simulink model "untitled_org"  (Simulink 10.0)
settings: Solver=ode45  StartTime=0.0  StopTime=10.0  RelTol=1e-3  EnableMultiTasking=on
undefined symbols (not defined in the file): water_level
libraries: nesl_utility x8, sm_lib x3
settings Model: Creator=Metti  LastModifiedBy=bhisma
settings DataIOCC: LimitDataPoints=on
settings OptimizationCC: ExpressionDepthLimit=2147483647
settings DebuggingCC: SolverPrmCheckMsg=warning  StateNameClashWarn=warning
settings GRTTargetCC: GeneratePreprocessorConditionals=Disable all  CombineOutputUpdateFcns=on  GRTInterface=off
settings ConfigComp: CovExternalEMLEnable=off
settings SimscapeCC: SimscapeNormalizeSystem=off
settings ConfigurationSet: Description=SimMechanics 2G

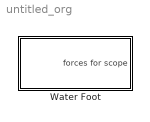
== system untitled_org ==
  Water Foot : Subsystem  AncestorBlock=WaterRunner_lib/Water Foot

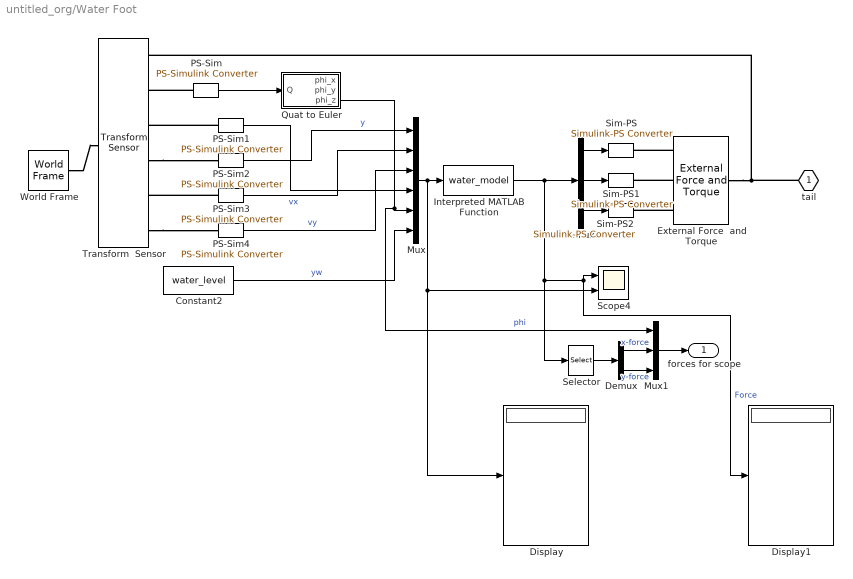
== system untitled_org/Water Foot ==
  Constant2 : Constant  Value=water_level
  Demux : Demux  Outputs=2
  Demux1 : Demux  Outputs=3
  Display : Display
  Display1 : Display
  External Force  and Torque : sm_lib/Forces and Torques/External Force and Torque  ForceResolutionFrame=World  EnableForceX=off  EnableForceY=on  EnableForceZ=on  EnableForce=off  TorqueResolutionFrame=World  EnableTorqueX=on  EnableTorqueY=off  EnableTorqueZ=off  EnableTorque=off
  Interpreted MATLAB Function : MATLABFcn  MATLABFcn=water_model
  Mux : Mux  Inputs=6
  Mux1 : Mux  Inputs=3
  PS-Sim{,1..4} (5 alike) : nesl_utility/PS-Simulink Converter  PhysicalDomain=network_engine_domain  SubClassName=ps_output  LeftPortType=input  RightPortType=output  PseudoPeriodic=off  Frequencies=[]  Unit=1  AffineConversion=off
  Quat to Euler : Subsystem
  Scope4 : Scope  NumInputPorts=2
  Selector : Selector  InputPortWidth=3  IndexOptions=Index vector (dialog)  Indices=[1 2]  OutputSizes=1
  Sim-PS : nesl_utility/Simulink-PS Converter  PhysicalDomain=network_engine_domain  SubClassName=ps_input  LeftPortType=input  RightPortType=output  PseudoPeriodic=off  Frequencies=[]  NoiseDistribution=none  NoiseParameters=[]  Unit=1  AffineConversion=off  FilteringAndDerivatives=zero  SimscapeFilterOrder=1  InputFilterTimeConstant=.001  UdotUserProvided=[]
  Sim-PS1 : nesl_utility/Simulink-PS Converter  PhysicalDomain=network_engine_domain  SubClassName=ps_input  LeftPortType=input  RightPortType=output  PseudoPeriodic=off  Frequencies=[]  NoiseDistribution=none  NoiseParameters=[]  Unit=1  AffineConversion=off  FilteringAndDerivatives=zero  SimscapeFilterOrder=1  InputFilterTimeConstant=.001  UdotUserProvided=[]
  Sim-PS2 : nesl_utility/Simulink-PS Converter  PhysicalDomain=network_engine_domain  SubClassName=ps_input  LeftPortType=input  RightPortType=output  PseudoPeriodic=off  Frequencies=[]  NoiseDistribution=none  NoiseParameters=[]  Unit=1  AffineConversion=off  FilteringAndDerivatives=zero  SimscapeFilterOrder=1  InputFilterTimeConstant=.001  UdotUserProvided=[]
  Transform  Sensor : sm_lib/Frames and Transforms/Transform Sensor  MeasurementFrame=World  SenseAngle=off  SenseAxis=off  SenseAngle1=off  SenseAngle2=off  SenseAngle3=off  SenseQ=on  SenseR=off  SenseOmegaX=off  SenseOmegaY=off  SenseOmegaZ=on  SenseOmega1=off  SenseOmega2=off  SenseOmega3=off  SenseQDot=off  SenseRDot=off  SenseAlphaX=off  SenseAlphaY=off  SenseAlphaZ=off  SenseAlpha1=off  SenseAlpha2=off  SenseAlpha3=off  SenseQDDot=off  SenseRDDot=off  SenseX=off  SenseY=on  SenseZ=off  SenseRad=off  SenseAzim=off  SenseDist=off  SenseInc=off  SenseXDot=on  SenseYDot=on  SenseZDot=off  SenseRadDot=off  SenseAzimDot=off  SenseDistDot=off  SenseIncDot=off  SenseXDDot=off  SenseYDDot=off  SenseZDDot=off  SenseRadDDot=off  SenseAzimDDot=off  SenseDistDDot=off  SenseIncDDot=off
  World Frame : sm_lib/Frames and Transforms/World Frame
  tail : PMIOPort  Side=Left
  forces for scope : Outport
  wires:
  Demux1/3 -> Sim-PS2/1
  Demux1/2 -> Sim-PS1/1
  Demux1/1 -> Sim-PS/1
  Mux/1 -> Scope4/2, Display/1, Interpreted MATLAB Function/1
  Interpreted MATLAB Function/1 -> Display1/1, Scope4/1, Selector/1, Demux1/1  "Force"
  Mux1/1 -> forces for scope/1
  Selector/1 -> Demux/1
  Demux/1 -> Mux1/2  "x-force"
  Demux/2 -> Mux1/3  "y-force"
  PS-Sim2/1 -> Mux/1  "y"
  PS-Sim3/1 -> Mux/2  "vx"
  PS-Sim4/1 -> Mux/3  "vy"
  PS-Sim1/1 -> Mux/4
  Constant2/1 -> Mux/6  "yw"
  PS-Sim/1 -> Quat to Euler/1(Q)
  Quat to Euler/3(phi_z) -> Mux1/1, Mux/5  "phi"
  connections:
  External Force  and Torque/LConn3 -- Sim-PS2/RConn1
  External Force  and Torque/LConn2 -- Sim-PS1/RConn1
  External Force  and Torque/LConn1 -- Sim-PS/RConn1
  Transform  Sensor/RConn6 -- PS-Sim4/LConn1
  PS-Sim3/LConn1 -- Transform  Sensor/RConn5
  Transform  Sensor/RConn4 -- PS-Sim2/LConn1
  PS-Sim1/LConn1 -- Transform  Sensor/RConn3
  PS-Sim/LConn1 -- Transform  Sensor/RConn2
  World Frame/RConn1 -- Transform  Sensor/LConn1
  External Force  and Torque/RConn1 -- tail/RConn1 -- Transform  Sensor/RConn1

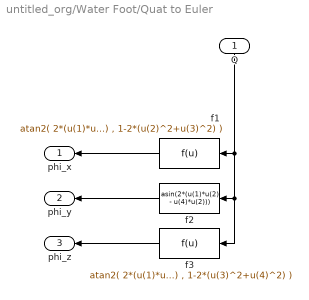
== system untitled_org/Water Foot/Quat to Euler ==
  Q : Inport
  f1 : Fcn  Expr=atan2( 2*(u(1)*u(2) + u(3)*u(4)) , 1-2*(u(2)^2+u(3)^2) )
  f2 : Fcn  Expr=asin(2*(u(1)*u(2) - u(4)*u(2)))
  f3 : Fcn  Expr=atan2( 2*(u(1)*u(4) + u(2)*u(3)) , 1-2*(u(3)^2+u(4)^2) )
  phi_x : Outport
  phi_y : Outport  Port=2
  phi_z : Outport  Port=3
  wires:
  Q/1 -> f3/1, f2/1, f1/1
  f1/1 -> phi_x/1
  f2/1 -> phi_y/1
  f3/1 -> phi_z/1
